simulink model "verify_T_Sensor_mdl"  (R2016b)
settings: Solver=ode45  StartTime=0.0  StopTime=100  MaxStep=1  RelTol=1e-3  EnableMultiTasking=on
libraries: carnot x3, simulink x1
settings Model: Creator=drhf  LastModifiedBy=drhf
settings DataIOCC: SaveFormat=Array  SignalLoggingSaveFormat=ModelDataLogs
settings OptimizationCC: ExpressionDepthLimit=2147483647  LifeSpan=inf
settings DebuggingCC: UnderspecifiedInitializationDetection=Classic  MergeDetectMultiDrivingBlocksExec=none  SolverPrmCheckMsg=warning  FcnCallInpInsideContextMsg=warning  StateNameClashWarn=warning  SFUnexpectedBacktrackingDiag=warning  SFNoUnconditionalDefaultTransitionDiag=warning  SFExecutionAtInitializationDiag=none
settings HardwareCC: ProdBitPerPointer=32  ProdBitPerSizeT=32  ProdBitPerPtrDiffT=32  ProdLargestAtomicFloat=None  ProdIntDivRoundTo=Undefined  ProdEndianess=Unspecified  ProdWordSize=32  ProdHWDeviceType=32-bit Generic
settings ModelReferenceCC: PropagateSignalLabelsOutOfModel=off
settings GRTTargetCC: TargetLangStandard=C89/C90 (ANSI)  GeneratePreprocessorConditionals=Disable all  CombineOutputUpdateFcns=off  GRTInterface=on
settings ConfigComp: CovMetricSettings=dw  CovHtmlReporting=on  CovSaveCumulativeToWorkspaceVar=on  CovSaveSingleToWorkspaceVar=on  CovExternalEMLEnable=off

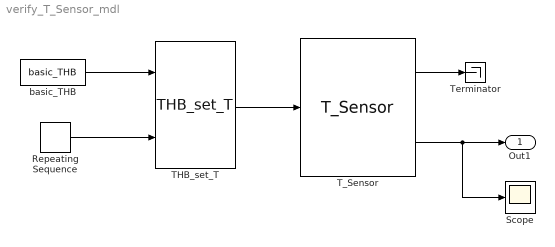
== system verify_T_Sensor_mdl ==
  Repeating Sequence : simulink/Sources/Repeating Sequence  rep_seq_t=[0 50 50.1 100]  rep_seq_y=[20 20 50 50]
  Scope : Scope
  THB_set_T : carnot/Source/Simple/THB_set_T
  T_Sensor : carnot/Control/T_Sensor  tc=5  t0=0
  Terminator : Terminator
  basic_THB : carnot/Basic/Hydraulics/basic_THB  t=70  mdot=200/3600  p=1e5  ID=Pressure Drop from Massflow  fluid=Water  mix=0  mix2=0  mix3=0  dia=0.02  hgt=0
  Out1 : Outport
  wires:
  T_Sensor/2 -> Scope/1, Out1/1
  basic_THB/1 -> THB_set_T/1
  T_Sensor/1 -> Terminator/1
  THB_set_T/1 -> T_Sensor/1
  Repeating Sequence/1 -> THB_set_T/2
